simulink model "AA2sfunc"  (R2021a)
settings: Solver=VariableStepAuto  StartTime=0.0  StopTime=200  RelTol=1e-3
libraries: simulink x1
settings Model: Creator=jhaid  LastModifiedBy=jhaid

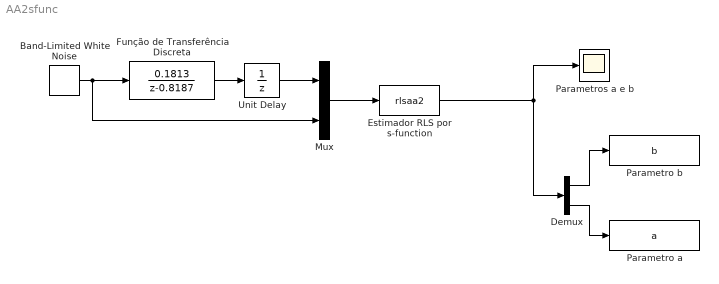
== system AA2sfunc ==
  Band-Limited White Noise : simulink/Sources/Band-Limited White Noise  Cov=[10]  Ts=20  seed=[23341]
  Demux : Demux  Outputs=2
  Estimador RLS por s-function : S-Function  FunctionName=rlsaa2  SFunctionDeploymentMode=off  EnableBusSupport=off
  Função de Transferência Discreta : DiscreteTransferFcn  Numerator=0.1813  Denominator="[1   -0.8187]"  InitialStates=1
  Mux : Mux  Inputs=2
  Parametro a : ToWorkspace  VariableName=a  SampleTime=-1
  Parametro b : ToWorkspace  VariableName=b  SampleTime=-1
  Parametros a e b : Scope
  Unit Delay : UnitDelay  SampleTime=-1  HasFrameUpgradeWarning=on
  wires:
  Mux/1 -> Estimador RLS por s-function/1
  Estimador RLS por s-function/1 -> Parametros a e b/1, Demux/1
  Demux/1 -> Parametro b/1
  Demux/2 -> Parametro a/1
  Função de Transferência Discreta/1 -> Unit Delay/1
  Unit Delay/1 -> Mux/1
  Band-Limited White Noise/1 -> Função de Transferência Discreta/1, Mux/2
